simulink model "model_opt_Matlab_2015a"  (R2015a)
settings: Solver=ode4  StartTime=0.0  StopTime=10.0  FixedStep=0.01  RelTol=1e-3
values from neighbouring files (symbols this model uses):
  alpha_0 = -1    [uczenie.m]
  b_nc = [0 0 0]'    [fuzzy_cel.m]    (also in uczenie.m)
  J = 1/3*2*0.4^2    (= 0.106666666667)    [dane.m]    (also in fuzzy_cel.m; uczenie.m)
  Ke = 10    [dane.m]    (also in fuzzy_cel.m; uczenie.m)
  L = 0.05    [dane.m]    (also in fuzzy_cel.m; uczenie.m)
  R = 10    [dane.m]    (also in fuzzy_cel.m; uczenie.m)
  sat_wsp1 = -2.65    [fuzzy_cel.m]    (also in uczenie.m)
  sat_wsp2 = -5.33    [fuzzy_cel.m]    (also in uczenie.m)
  U_g1 = 0.5    [fuzzy_cel.m]    (also in uczenie.m)
  U_g2 = 1    [fuzzy_cel.m]    (also in uczenie.m)
  W = [kd1 kp1 ki1 0 ... (first row only)    [fuzzy_cel.m]    (also in uczenie.m)
  z_max = 1    [fuzzy_cel.m]    (also in uczenie.m)
  z_min = -1    [fuzzy_cel.m]    (also in uczenie.m)
undefined symbols (not defined in the file or in its folder): sigbuilder_block
settings Model: Creator=Student  LastModifiedBy=Maciek

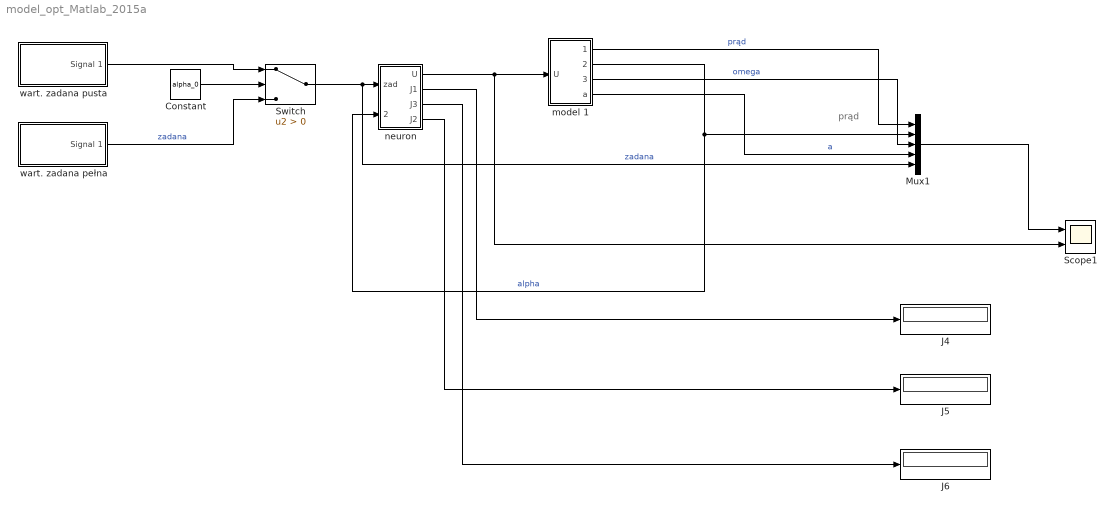
== system model_opt_Matlab_2015a ==
  note: prąd
  Constant : Constant  Value=alpha_0
  J4 : Display
  J5 : Display
  J6 : Display
  Mux1 : Mux  Inputs=5
  Scope1 : Scope  NumInputPorts=2
      settings: TimeRange=auto  ShowLegends=on  MaxDataPoints=5000  YMin=-11.15117~-1.19117  YMax=6.61807~0.72057  SampleTime=-1
  Switch : Switch  Criteria=u2 > Threshold
  model 1 : Subsystem
  neuron : Subsystem
  wart. zadana pełna : Subsystem  Tag=STV Subsys  LoadFcn=sigbuilder_block('load');  StartFcn=sigbuilder_block('start');  StopFcn=sigbuilder_block('stop');  ClipboardFcn=sigbuilder_block('clipboard');  mask(Sigbuilder block){}
      mask help: Simulink:masks:SigbuilderBlock_MD
      mask init:
      | if ~strcmp(get_param(bdroot(gcbh),'SimulationStatus'),'stopped') tuvar = sigbuilder_block('maskInit'); end
      settings: CopyFcn=sigbuilder_block('copy');  DeleteFcn=sigbuilder_block('delete');  ModelCloseFcn=sigbuilder_block('modelClose');  PreSaveFcn=sigbuilder_block('preSave');  PauseFcn=sigbuilder_block('pause');  ContinueFcn=sigbuilder_block('continue');  NameChangeFcn=sigbuilder_block('namechange');  OpenFcn=sigbuilder_block('open',[437.25 153.75 550.5 359.25 ]);  CloseFcn=sigbuilder_block('close');
      mask Display: plot(0, 0, 100, 100,[2, 2, 32, 32, 2], [68, 8, 8, 68, 68],[32, 2], [38, 38], [32, 19, 2],[53, 60, 44], [32, 17, 17, 2],[16, 16, 31, 31]);txt = getActiveGroup(gcbh);text(2, 100, txt,'verticalAlignment', 'top');
  wart. zadana pusta : Subsystem  Tag=STV Subsys  LoadFcn=sigbuilder_block('load');  StartFcn=sigbuilder_block('start');  StopFcn=sigbuilder_block('stop');  ClipboardFcn=sigbuilder_block('clipboard');  mask(Sigbuilder block){}
      mask help: Simulink:masks:SigbuilderBlock_MD
      mask init:
      | if ~strcmp(get_param(bdroot(gcbh),'SimulationStatus'),'stopped') tuvar = sigbuilder_block('maskInit'); end
      settings: CopyFcn=sigbuilder_block('copy');  DeleteFcn=sigbuilder_block('delete');  ModelCloseFcn=sigbuilder_block('modelClose');  PreSaveFcn=sigbuilder_block('preSave');  PauseFcn=sigbuilder_block('pause');  ContinueFcn=sigbuilder_block('continue');  NameChangeFcn=sigbuilder_block('namechange');  OpenFcn=sigbuilder_block('open',[437.25 153.75 550.5 359.25 ]);  CloseFcn=sigbuilder_block('close');
      mask Display: plot(0, 0, 100, 100,[2, 2, 32, 32, 2], [68, 8, 8, 68, 68],[32, 2], [38, 38], [32, 19, 2],[53, 60, 44], [32, 17, 17, 2],[16, 16, 31, 31]);txt = getActiveGroup(gcbh);text(2, 100, txt,'verticalAlignment', 'top');
  wires:
  neuron/2(J1) -> J4/1
  neuron/3("J3 ") -> J6/1
  neuron/4("J2 ") -> J5/1
  Mux1/1 -> Scope1/1
  Switch/1 -> Mux1/5, neuron/1(zad)  "zadana"
  model 1/2(alpha) -> Mux1/2, neuron/2(alpha)  "alpha"
  model 1/1(prąd) -> Mux1/1  "prąd"
  model 1/3(omega) -> Mux1/3  "omega"
  model 1/4(a) -> Mux1/4  "a"
  neuron/1(U) -> model 1/1(U), Scope1/2
  Constant/1 -> Switch/2
  wart. zadana pusta/1(Signal 1) -> Switch/1
  wart. zadana pełna/1(Signal 1) -> Switch/3  "zadana"

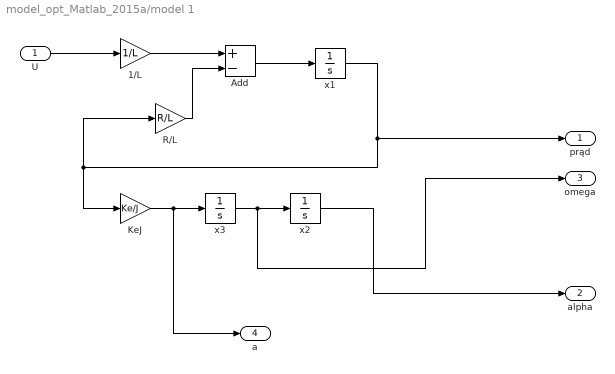
== system model_opt_Matlab_2015a/model 1 ==
  U : Inport
  "1/L " : Gain  Gain=1/L
  Add : Sum  Inputs=+-
  KeJ : Gain  Gain=Ke/J
  R/L : Gain  Gain=R/L
  "x1 " : Integrator
  x2 : Integrator  InitialCondition=alpha_0
  "x3 " : Integrator
  prąd : Outport
  alpha : Outport  Port=2
  omega : Outport  Port=3
  a : Outport  Port=4
  wires:
  U/1 -> "1/L "/1
  x2/1 -> alpha/1
  KeJ/1 -> a/1, "x3 "/1
  "x3 "/1 -> omega/1, x2/1
  Add/1 -> "x1 "/1
  "1/L "/1 -> Add/1
  R/L/1 -> Add/2
  "x1 "/1 -> KeJ/1, R/L/1, prąd/1

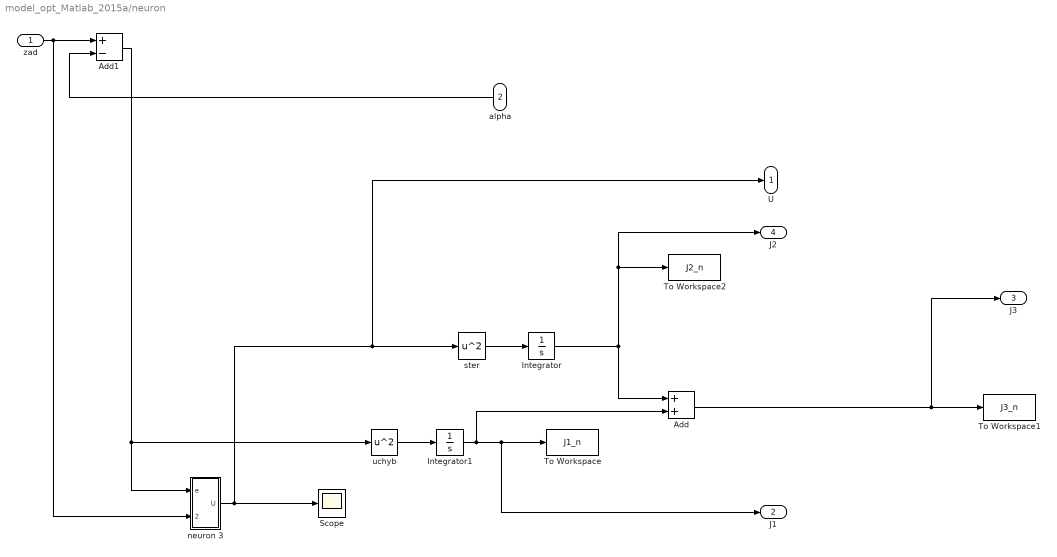
== system model_opt_Matlab_2015a/neuron ==
  zad : Inport
  alpha : Inport  Port=2
  Add : Sum
  Add1 : Sum  Inputs=+-
  Integrator : Integrator
  Integrator1 : Integrator
  Scope : Scope
      settings: TimeRange=auto  MaxDataPoints=5000  SaveToWorkspace=off  SaveName=ScopeData2  YMin=-1.237  YMax=1.13298  SampleTime=-1
  To Workspace : ToWorkspace  VariableName=J1_n  SampleTime=-1
      settings: MaxDataPoints=1
  To Workspace1 : ToWorkspace  VariableName=J3_n  SampleTime=-1
      settings: MaxDataPoints=1
  To Workspace2 : ToWorkspace  VariableName=J2_n  SampleTime=-1
      settings: MaxDataPoints=1
  neuron 3 : Subsystem
  ster : Math  Operator=square  SaturateOnIntegerOverflow=on
  "uchyb " : Math  Operator=square  SaturateOnIntegerOverflow=on
  U : Outport
  J1 : Outport  Port=2
  "J3 " : Outport  Port=3
  "J2 " : Outport  Port=4
  wires:
  alpha/1 -> Add1/2
  zad/1 -> neuron 3/2(zad), Add1/1
  Add1/1 -> neuron 3/1(e), "uchyb "/1
  ster/1 -> Integrator/1
  "uchyb "/1 -> Integrator1/1
  Integrator1/1 -> Add/2, J1/1, To Workspace/1
  Integrator/1 -> To Workspace2/1, "J2 "/1, Add/1
  Add/1 -> "J3 "/1, To Workspace1/1
  neuron 3/1("U ") -> U/1, ster/1, Scope/1

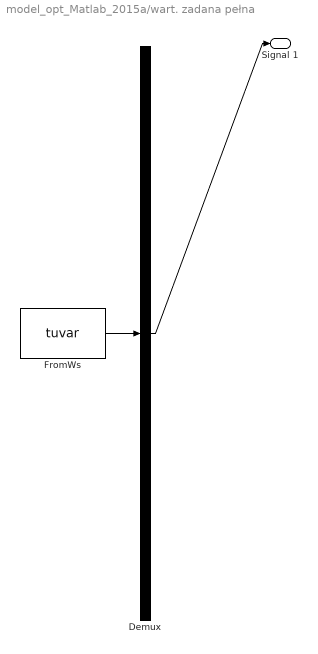
== system model_opt_Matlab_2015a/wart. zadana pełna ==
  Demux : Demux  Tag=STV Demux  Outputs=1
  FromWs : FromWorkspace  Tag=STV FromWs  VariableName=tuvar  SampleTime=0
      SigBuilderData=|
      | common.afterFinalStr = 'Extrapolate'
      | common.sampleTime = 0
      | dataSet.timeRange = [0 10]
      | dataSet.name = 'Group 1'
      | sbobj.Groups.Name = 'Group 1'
      | sbobj.Groups.Signals.Name = 'Signal 1'
      | sbobj.Groups.Signals.XData = [0 3 3 5 5 8 8 10]
      | sbobj.Groups.Signals.YData = [1 1 -1 -1 1 1 -1 -1]
  Signal 1 : Outport  Tag=STV Outport
  wires:
  FromWs/1 -> Demux/1
  Demux/1 -> Signal 1/1

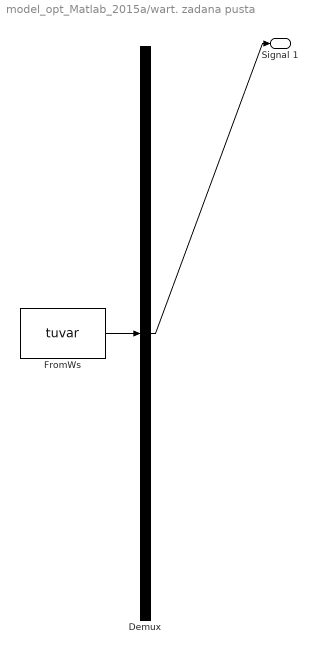
== system model_opt_Matlab_2015a/wart. zadana pusta ==
  Demux : Demux  Tag=STV Demux  Outputs=1
  FromWs : FromWorkspace  Tag=STV FromWs  VariableName=tuvar  SampleTime=0
      SigBuilderData=|
      | common.afterFinalStr = 'Extrapolate'
      | common.sampleTime = 0
      | dataSet.timeRange = [0 10]
      | dataSet.name = 'Group 1'
      | sbobj.Groups.Name = 'Group 1'
      | sbobj.Groups.Signals.Name = 'Signal 1'
      | sbobj.Groups.Signals.XData = [0 2 2 5 5 8 8 10]
      | sbobj.Groups.Signals.YData = [-1 -1 1 1 -1 1 -1 -1]
  Signal 1 : Outport  Tag=STV Outport
  wires:
  Demux/1 -> Signal 1/1
  FromWs/1 -> Demux/1

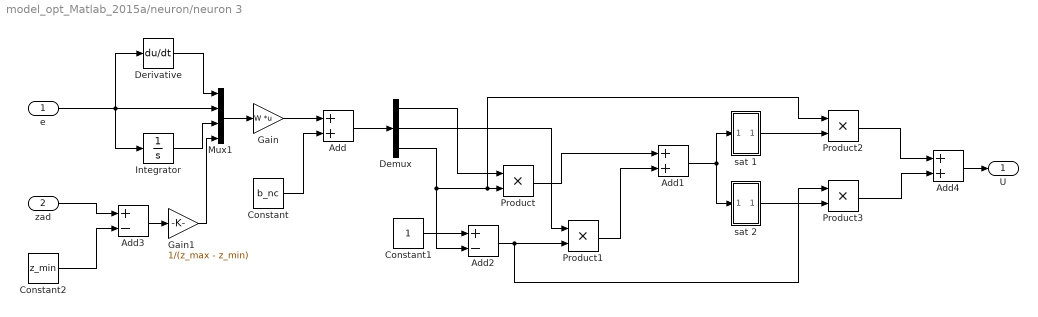
== system model_opt_Matlab_2015a/neuron/neuron 3 ==
  e : Inport
  zad : Inport  Port=2
  Add : Sum
  Add1 : Sum
  Add2 : Sum  Inputs=+-
  Add3 : Sum  Inputs=+-
  Add4 : Sum
  Constant : Constant  Value=b_nc
  Constant1 : Constant
  Constant2 : Constant  Value=z_min
  Demux : Demux  Outputs=3
  Derivative : Derivative
  Gain : Gain  Gain=W  Multiplication=Matrix(K*u) (u vector)
  Gain1 : Gain  Gain=1/(z_max - z_min)
  Integrator : Integrator
  Mux1 : Mux
  Product{,1..3} (4 alike) : Product
  sat 1 : Subsystem
  sat 2 : Subsystem
  "U " : Outport
  wires:
  Integrator/1 -> Mux1/3
  e/1 -> Integrator/1, Derivative/1, Mux1/2
  Derivative/1 -> Mux1/1
  Gain/1 -> Add/1
  Constant/1 -> Add/2
  Mux1/1 -> Gain/1
  Add1/1 -> sat 2/1(in), sat 1/1(in)
  Add/1 -> Demux/1
  Demux/2 -> Product1/1
  Demux/1 -> Product/1
  Demux/3 -> Add2/2, Product2/1, Product/2
  Product/1 -> Add1/1
  Constant1/1 -> Add2/1
  Add2/1 -> Product3/1, Product1/2
  Product1/1 -> Add1/2
  Add3/1 -> Gain1/1
  zad/1 -> Add3/1
  Constant2/1 -> Add3/2
  sat 1/1(u) -> Product2/2
  sat 2/1(u) -> Product3/2
  Product2/1 -> Add4/1
  Product3/1 -> Add4/2
  Add4/1 -> "U "/1
  Gain1/1 -> Mux1/4

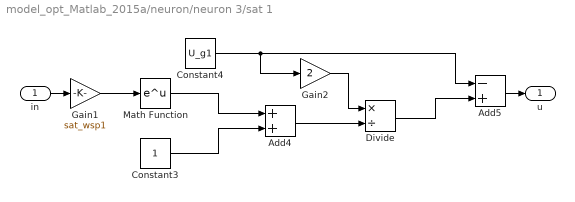
== system model_opt_Matlab_2015a/neuron/neuron 3/sat 1 ==
  in : Inport
  Add4 : Sum
  Add5 : Sum  Inputs=-+
  Constant3 : Constant
  Constant4 : Constant  Value=U_g1
  Divide : Product  Inputs=*/
  Gain1 : Gain  Gain=sat_wsp1
  Gain2 : Gain  Gain=2
  Math Function : Math  SaturateOnIntegerOverflow=on
  u : Outport
  wires:
  Divide/1 -> Add5/2
  Math Function/1 -> Add4/1
  Constant4/1 -> Gain2/1, Add5/1
  Gain1/1 -> Math Function/1
  Gain2/1 -> Divide/1
  Add4/1 -> Divide/2
  Constant3/1 -> Add4/2
  in/1 -> Gain1/1
  Add5/1 -> u/1

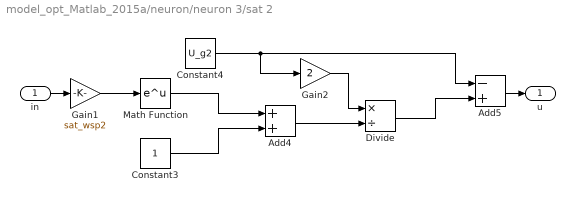
== system model_opt_Matlab_2015a/neuron/neuron 3/sat 2 ==
  in : Inport
  Add4 : Sum
  Add5 : Sum  Inputs=-+
  Constant3 : Constant
  Constant4 : Constant  Value=U_g2
  Divide : Product  Inputs=*/
  Gain1 : Gain  Gain=sat_wsp2
  Gain2 : Gain  Gain=2
  Math Function : Math  SaturateOnIntegerOverflow=on
  u : Outport
  wires:
  Divide/1 -> Add5/2
  Math Function/1 -> Add4/1
  Constant4/1 -> Gain2/1, Add5/1
  Gain1/1 -> Math Function/1
  Gain2/1 -> Divide/1
  Add4/1 -> Divide/2
  Constant3/1 -> Add4/2
  in/1 -> Gain1/1
  Add5/1 -> u/1
